simulink model "sim_TCC_2024"  (R2024b)
settings: Solver=FixedStepAuto  StartTime=0.0  StopTime=Tsim  FixedStep=Ts_sim  RelTol=1e-3
InitFcn:
  | traj
values from neighbouring files (symbols this model uses):
  dist = 0.1 * Lim_Torque_motor * [1, 1, 1]    [main_automacao.m]    (also in main_run.m = [0.5*Lim_Torque_motor,0.5*Lim_Torque_motor,0.5*Lim_Torque_mo)
  DISTURBANCE_ON = 1    [main_automacao.m]    (also in main_run.m)
  end_learning_time = 5 * Tspan    (= 50)    [main_automacao.m]    (also in main_run.m)
  error_difference = [ ... (first row only)    [main_automacao.m]    (also in main_run.m = [r(1),0,r(2),0,r(3),0])
  IC_ERROR_ON = 1    [main_automacao.m]    (also in main_run.m = 0)
  ILC_ON = method.ILC_ON    [main_automacao.m]    (also in main_run.m = 1)
  Kp0 = gains(1)    [main_automacao.m]    (also in main_run.m = 30)
  Kp1 = gains(3)    [main_automacao.m]    (also in main_run.m = 30)
  Kp2 = gains(5)    [main_automacao.m]    (also in main_run.m = 30)
  Kv0 = gains(2)    [main_automacao.m]    (also in main_run.m = 2.5)
  Kv1 = gains(4)    [main_automacao.m]    (also in main_run.m = 2.5)
  Kv2 = gains(6)    [main_automacao.m]    (also in main_run.m = 2.5)
  Lim_Torque_motor = 1.4    [main_automacao.m]    (also in main_run.m = 1)
  m_payload = 0.125    [main_automacao.m]    (also in main_run.m)
  NOISE_ON = 1    [main_automacao.m]    (also in main_run.m = 0)
  noise_power = [ ... (first row only)    [main_automacao.m]    (also in main_run.m = [1e-10,1e-10,1e-10,1e-10,1e-10,1e-10])
  PAYLOAD_ON = 1    [main_automacao.m]    (also in main_run.m = 0)
  SATURATION_ON = 1    [main_automacao.m]    (also in main_run.m)
  shift_time = Tspan / 2    (= 5)    [main_automacao.m]    (also in main_run.m; plot_trajetorias.m)
  t0_dist = end_learning_time + 2    (= 52)    [main_automacao.m]    (also in main_run.m = 26)
  t_pick = 0:Ts:Tspan/2-Ts    [main_automacao.m]    (also in main_run.m; plot_trajetorias.m = 0:Ts:cycle_duration/2-Ts)
  t_return = 0:Ts:Tspan/2-Ts    [main_automacao.m]    (also in main_run.m; plot_trajetorias.m = 0:Ts:cycle_duration/2-Ts)
  tf_dist = t0_dist + 2    (= 54)    [main_automacao.m]    (also in main_run.m = 32)
  Ts = 0.01    [main_automacao.m]    (also in main_run.m; plot_trajetorias.m)
  Tspan = 10    [main_automacao.m]    (also in main_run.m)
undefined symbols (not defined in the file or in its folder): q0_ida, q1_ida, q2_ida, qd0_ida, qd1_ida, qd2_ida, qdd0_ida, qdd1_ida, qdd2_ida
libraries: simulink x23, simulink_extras x3
settings Model: Creator=iury  LastModifiedBy=gabri
settings SolverCC: AlgebraicLoopSolver=TrustRegion
settings DataIOCC: ReturnWorkspaceOutputs=off
settings DebuggingCC: UnconnectedInputMsg=warning  UnconnectedOutputMsg=warning  UnconnectedLineMsg=warning  ArithmeticOperatorsInVariantConditions=warning
settings ModelReferenceCC: EnableRefExpFcnMdlSchedulingChecks=on
settings SFSimCC: SimUseLocalCustomCode=off  CustomCodeUndefinedFunction=UseInterfaceOnly
settings RTWCC: RTWUseLocalCustomCode=off  GPUComputeCapability=3.5
settings CodeAppCC: StateflowObjectComments=on
settings SimscapeCC: SimscapeNormalizeSystem=off

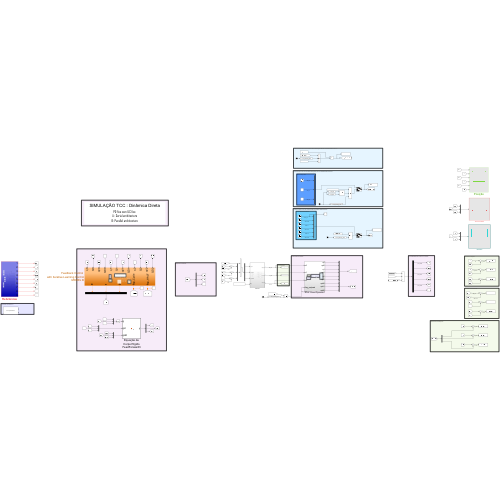
[thumbnail: Simulink's stored preview of the top-level diagram]
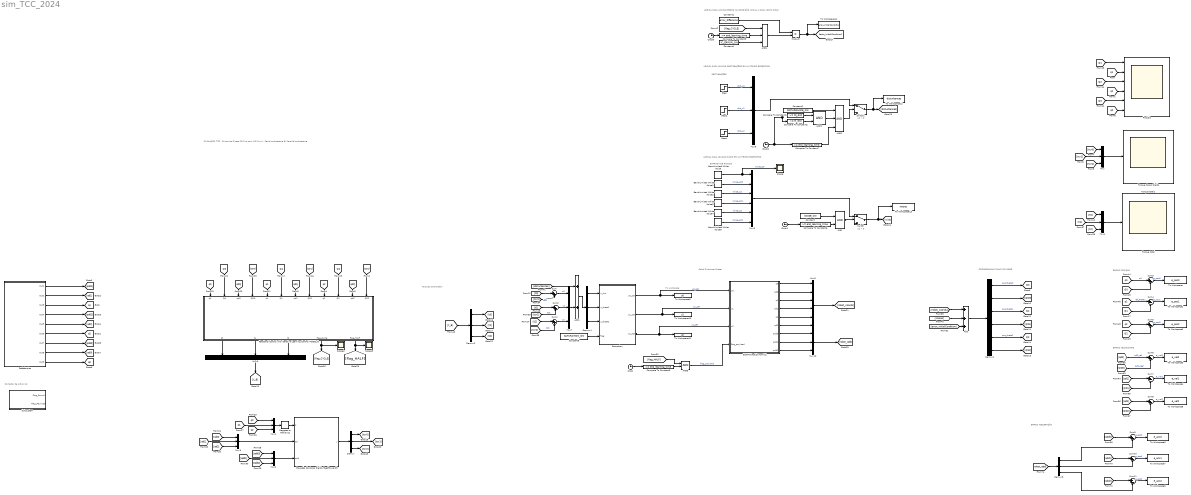
== system sim_TCC_2024 ==
  note: LÓGICA PARA APLICAR ERROS NA CONDIÇÃO INICIAL A CADA NOVO CICLO
  note: Contador de ciclos ILC
  note: PERTUBAÇÕES
  note: Torques controlador
  note: LÓGICA PARA APLICAR PERTUBAÇÕES EM UM TEMPO ESPECÍFICO
  note: Robô Dinâmica Direta
  note: COORDENADAS FINAIS DO ROBÔ
  note: ENTRADA DE RUÍDOS
  note: LÓGICA PARA APLICAR RUÍDO EM UM TEMPO ESPECÍFICO
  note: SIMULAÇÃO TCC : Dinâmica Direta
      |
      | PD fixo com ILC fixo
      | A : Serial architecture
      | B: Parallel architecture
  note: ERROS POSIÇAO
  note: ERROS VELOCIDADE
  note: ERROS ACELERAÇÃO
  note: To workspace
  3DOF Direct Dynamic1 : Subsystem
  AND : Logic  AllPortsSameDT=off  OutDataTypeStr=boolean
  AND1 : Logic  Inputs=3  AllPortsSameDT=off  OutDataTypeStr=boolean
  AND2 : Logic  AllPortsSameDT=off  OutDataTypeStr=boolean
  AND4 : Logic  Inputs=3  AllPortsSameDT=off  OutDataTypeStr=boolean
  AND5 : Logic  AllPortsSameDT=off  OutDataTypeStr=boolean
  Add : Sum  Inputs=+++
  Add1 : Sum
  Band-Limited White Noise : simulink/Sources/Band-Limited White Noise  Cov=noise_power(1)  Ts=Ts  seed=[1]
  Band-Limited White Noise1 : simulink/Sources/Band-Limited White Noise  Cov=noise_power(2)  Ts=Ts  seed=[2]
  Band-Limited White Noise2 : simulink/Sources/Band-Limited White Noise  Cov=noise_power(3)  Ts=Ts  seed=[3]
  Band-Limited White Noise3 : simulink/Sources/Band-Limited White Noise  Cov=noise_power(4)  Ts=Ts  seed=[4]
  Band-Limited White Noise4 : simulink/Sources/Band-Limited White Noise  Cov=noise_power(5)  Ts=Ts  seed=[5]
  Band-Limited White Noise5 : simulink/Sources/Band-Limited White Noise  Cov=noise_power(6)  Ts=Ts  seed=[6]
  Clock{,1..3} (4 alike) : Clock
  Compare To Constant1 : simulink/Logic and Bit Operations/Compare To Constant  relop=>=  const=t0_dist  OutDataTypeStr=boolean
  Compare To Constant2 : simulink/Logic and Bit Operations/Compare To Constant  relop=<=  const=tf_dist  OutDataTypeStr=boolean
  Compare To Constant{3,5..7} (4 alike) : simulink/Logic and Bit Operations/Compare To Constant  relop=>=  const=end_learning_time  OutDataTypeStr=boolean
  Constant : Constant  Value=NOISE_ON
  Constant1 : Constant  Value=error_difference
  Constant2 : Constant  Value=DISTURBANCE_ON
  Constant4 : Constant  Value=IC_ERROR_ON
  Constant5 : Constant  Value=SATURATION_ON
  Degrees to Radians2 : simulink_extras/Transformations/Degrees to Radians
  Demux{,2..4} (4 alike) : Demux  Outputs=3
  Demux1 : Demux  Outputs=6
  Equação de Corpo Rígido FeedForward3 : MATLAB Function  TreatAsAtomicUnit=on
  Feedback Control with Iterative Learning Control MODEL B : Subsystem
  Mux{,1..4,6..7,9..10} (9 alike) : Mux  Inputs=3
  Mux5 : Mux  Inputs=6
  Mux8 : Mux  Inputs=6
  Posição : Scope  NumInputPorts=6
  Product : Product
  Referências : Subsystem
  Saturation : Subsystem
  Scope : Scope
  Scope2 : Scope
  Scope3 : Scope
  Step : Step  After=dist(1)  SampleTime=Ts
  Step2 : Step  After=dist(2)  SampleTime=Ts
  Step4 : Step  After=dist(3)  SampleTime=Ts
  Subsystem : Subsystem  mask{Tspan=Tspan, Parameter3=Ts}
      mask prompts: Parameter3 "Sample Time"
      mask Display: disp('ILC Cycle Counter');
  Sum : Sum  Inputs=|++
  Sum1 : Sum  Inputs=|++
  Sum{3..11} (9 alike) : Sum  Inputs=|+-
  Sum2 : Sum  Inputs=|++
  Switch : Switch  Criteria=u2 > Threshold  SaturateOnIntegerOverflow=off  InputSameDT=off
  Switch1 : Switch  Criteria=u2 > Threshold  SaturateOnIntegerOverflow=off  InputSameDT=off
  To Workspace : ToWorkspace  VariableName=e_pos0  SaveFormat=Timeseries  SampleTime=-1
  To Workspace1 : ToWorkspace  VariableName=e_pos1  SaveFormat=Timeseries  SampleTime=-1
  To Workspace10 : ToWorkspace  VariableName=u1  SaveFormat=Timeseries  SampleTime=-1
  To Workspace11 : ToWorkspace  VariableName=u2  SaveFormat=Timeseries  SampleTime=-1
  To Workspace12 : ToWorkspace  VariableName=disturbances  SaveFormat=Timeseries  SampleTime=-1
  To Workspace13 : ToWorkspace  VariableName=noises  SaveFormat=Timeseries  SampleTime=-1
  To Workspace14 : ToWorkspace  VariableName=error_initialCondition  SaveFormat=Timeseries  SampleTime=-1
  To Workspace2 : ToWorkspace  VariableName=e_pos2  SaveFormat=Timeseries  SampleTime=-1
  To Workspace3 : ToWorkspace  VariableName=e_vel0  SaveFormat=Timeseries  SampleTime=-1
  To Workspace4 : ToWorkspace  VariableName=e_vel1  SaveFormat=Timeseries  SampleTime=-1
  To Workspace5 : ToWorkspace  VariableName=e_vel2  SaveFormat=Timeseries  SampleTime=-1
  To Workspace6 : ToWorkspace  VariableName=e_acc0  SaveFormat=Timeseries  SampleTime=-1
  To Workspace7 : ToWorkspace  VariableName=e_acc1  SaveFormat=Timeseries  SampleTime=-1
  To Workspace8 : ToWorkspace  VariableName=e_acc2  SaveFormat=Timeseries  SampleTime=-1
  To Workspace9 : ToWorkspace  VariableName=u0  SaveFormat=Timeseries  SampleTime=-1
  Torque Corpo Rígido : Scope
  Torque total : Scope
  Torque total1 : Scope
  tag scope: Q0=global, Q1=global, Q2=global, q0=global, q1=global, q2=global
  wires:
  Mux/1 -> Torque Corpo Rígido/1
  [q0] -> Feedback Control with Iterative Learning Control MODEL B/1(q0)
  [Q0] -> Feedback Control with Iterative Learning Control MODEL B/2(Q0)
  [qd0] -> Feedback Control with Iterative Learning Control MODEL B/3(qd0)
  [QD0] -> Feedback Control with Iterative Learning Control MODEL B/4(QD0)
  [q1] -> Feedback Control with Iterative Learning Control MODEL B/5(q1)
  [Q1] -> Feedback Control with Iterative Learning Control MODEL B/6(Q1)
  [qd1] -> Feedback Control with Iterative Learning Control MODEL B/7(qd1)
  [QD1] -> Feedback Control with Iterative Learning Control MODEL B/8(QD1)
  [q2] -> Feedback Control with Iterative Learning Control MODEL B/9(q2)
  [Q2] -> Feedback Control with Iterative Learning Control MODEL B/10(Q2)
  [QD2] -> Feedback Control with Iterative Learning Control MODEL B/12(QD2)
  [qd2] -> Feedback Control with Iterative Learning Control MODEL B/11(qd2)
  [Q1] -> Posição/1
  [q1] -> Posição/2
  [Q2] -> Posição/3
  [q2] -> Posição/4
  [Q0] -> Posição/5
  [q0] -> Posição/6
  Mux1/1 -> Degrees to Radians2/1
  [q0] -> Mux1/1
  [q2] -> Mux1/3
  [q1] -> Mux1/2
  [qdd0] -> Mux2/1
  [qdd2] -> Mux2/3
  [qdd1] -> Mux2/2
  [qd2] -> Mux3/3
  [qd1] -> Mux3/2
  [qd0] -> Mux3/1
  Demux/1 -> [tcr0]
  Demux/3 -> [tcr2]
  Demux/2 -> [tcr1]
  Equação de Corpo Rígido FeedForward3/1(y) -> Demux/1
  Mux3/1 -> Equação de Corpo Rígido FeedForward3/2(qd)
  Mux2/1 -> Equação de Corpo Rígido FeedForward3/3(qdd)
  Degrees to Radians2/1 -> Equação de Corpo Rígido FeedForward3/1(q)
  [tcr0] -> Mux/1
  [tcr1] -> Mux/2
  [tcr2] -> Mux/3
  [t1] -> Mux4/2
  Mux4/1 -> Torque total/1
  [t2] -> Mux4/3
  [t0] -> Mux4/1
  Feedback Control with Iterative Learning Control MODEL B/2(t1) -> Mux9/2
  Feedback Control with Iterative Learning Control MODEL B/3(t2) -> Mux9/3
  Feedback Control with Iterative Learning Control MODEL B/1(t0) -> Mux9/1
  [t0] -> Sum/1
  [t2] -> Sum1/1
  [t1] -> Sum2/1
  [tcr0] -> Sum/2  "tcr0"
  [tcr2] -> Sum1/2  "tcr2"
  [tcr1] -> Sum2/2  "tcr1"
  Band-Limited White Noise/1 -> Scope/1, Mux5/1  "noise_q0"
  Band-Limited White Noise1/1 -> Mux5/2  "noise_qd0"
  Band-Limited White Noise2/1 -> Mux5/3  "noise_q1"
  Band-Limited White Noise3/1 -> Mux5/4  "noise_qd1"
  Band-Limited White Noise4/1 -> Mux5/5  "noise_q2"
  Band-Limited White Noise5/1 -> Mux5/6  "noise_qd2"
  Mux5/1 -> Switch/1
  Demux1/1 -> [Q0]  "pos_theta0"
  Demux1/2 -> [QD0]
  Demux1/3 -> [Q1]  "pos_theta1"
  Demux1/4 -> [QD1]
  Demux1/5 -> [Q2]  "pos_theta2"
  Demux1/6 -> [QD2]
  Add/1 -> Demux1/1
  Constant/1 -> AND/1
  AND/1 -> Switch/2
  3DOF Direct Dynamic1/1(q0) -> Mux8/1
  3DOF Direct Dynamic1/2(qd0) -> Mux8/2
  3DOF Direct Dynamic1/3(q1) -> Mux8/3
  3DOF Direct Dynamic1/4(qd1) -> Mux8/4
  3DOF Direct Dynamic1/5(q2) -> Mux8/5
  3DOF Direct Dynamic1/6(qd2) -> Mux8/6
  Step/1 -> Mux6/1  "dist_u0"
  Step2/1 -> Mux6/2  "dist_u1"
  Step4/1 -> Mux6/3  "dist_u2"
  AND1/1 -> Switch1/2
  Constant2/1 -> AND1/1
  Compare To Constant1/1 -> AND2/1
  Compare To Constant2/1 -> AND2/2
  Clock2/1 -> Compare To Constant2/1, Compare To Constant1/1, Compare To Constant7/1
  Mux6/1 -> Switch1/1
  Switch1/1 -> To Workspace12/1, [disturbances]
  Switch/1 -> To Workspace13/1, [noises]
  Mux9/1 -> [t_B]
  [t_B] -> Demux2/1
  Demux2/1 -> [t0]
  Demux2/2 -> [t1]
  Demux2/3 -> [t2]
  [q0] -> Sum3/1  "q0"
  Sum3/1 -> To Workspace/1  "e_pos0"
  [q2] -> Sum5/1
  [Q1] -> Sum4/2
  [Q2] -> Sum5/2
  [Q0] -> Sum3/2
  [q1] -> Sum4/1  "ref_theta1"
  Sum4/1 -> To Workspace1/1  "e_pos1"
  Sum5/1 -> To Workspace2/1  "e_pos2"
  Sum7/1 -> To Workspace4/1  "e_vel1"
  [QD1] -> Sum7/2
  [qd1] -> Sum7/1
  [qd0] -> Sum6/1  "qd0_ref"
  [QD2] -> Sum8/2
  Sum6/1 -> To Workspace3/1  "e_vel0"
  [qd2] -> Sum8/1
  [QD0] -> Sum6/2  "qd0_real"
  Sum8/1 -> To Workspace5/1  "e_vel2"
  Sum10/1 -> To Workspace7/1  "e_acc1"
  [qdd1] -> Sum10/1
  Sum11/1 -> To Workspace8/1  "e_acc2"
  [qdd0] -> Sum9/1
  Demux3/2 -> Sum10/2
  Demux3/1 -> Sum9/2
  Sum9/1 -> To Workspace6/1  "e_acc0"
  Demux3/3 -> Sum11/2
  [qdd2] -> Sum11/1
  3DOF Direct Dynamic1/7(qdd0) -> Mux10/1
  3DOF Direct Dynamic1/8(qdd1) -> Mux10/2
  3DOF Direct Dynamic1/9(qdd2) -> Mux10/3
  Mux10/1 -> [robot_qdd]
  [robot_qdd] -> Demux3/1
  [robot_coords] -> Add/1
  [noises] -> Add/2
  [flag_CYCLE] -> AND4/1
  [error_initialCondition] -> Add/3
  Constant4/1 -> AND4/3
  Referências/1(Out1) -> [qdd1]
  Referências/2(Out2) -> [qd1]
  Referências/3(Out3) -> [q1]
  Referências/4(Out4) -> [qdd2]
  Referências/5(Out5) -> [qd2]
  Referências/6(Out6) -> [q2]
  Referências/7(Out7) -> [qdd0]
  Referências/8(Out8) -> [qd0]
  Referências/9(Out9) -> [q0]
  Mux8/1 -> [robot_coords]
  Saturation/1(u0_sat) -> 3DOF Direct Dynamic1/1(u0), To Workspace9/1  "u0_sat"
  Saturation/2(u1_sat) -> To Workspace10/1, 3DOF Direct Dynamic1/2(u1)  "u1_sat"
  Saturation/3(u2_sat) -> 3DOF Direct Dynamic1/3(u2), To Workspace11/1  "u2_sat"
  Constant5/1 -> Saturation/4(flag)
  Sum2/1 -> Mux7/2  "u1"
  Sum/1 -> Mux7/1  "u0"
  Sum1/1 -> Mux7/3  "u2"
  [disturbances] -> Add1/1
  Mux7/1 -> Add1/2
  Add1/1 -> Demux4/1
  Demux4/1 -> Saturation/1(u_rho)
  Demux4/2 -> Saturation/2(u_theta1)
  Demux4/3 -> Saturation/3(u_theta2)
  AND2/1 -> AND1/2
  [flag_HALF] -> AND5/1
  AND5/1 -> 3DOF Direct Dynamic1/4(flag_payload)  "flag_payload"
  Clock/1 -> Compare To Constant5/1
  Compare To Constant5/1 -> AND5/2
  Feedback Control with Iterative Learning Control MODEL B/4(flag_Cycle) -> Scope2/1, [flag_CYCLE]
  Feedback Control with Iterative Learning Control MODEL B/5(flag_HALF) -> Scope3/1, [flag_HALF]
  Clock1/1 -> Compare To Constant6/1
  Compare To Constant6/1 -> AND/2
  Compare To Constant7/1 -> AND1/3
  Compare To Constant3/1 -> AND4/2
  Clock3/1 -> Compare To Constant3/1
  AND4/1 -> Product/2
  Constant1/1 -> Product/1
  Product/1 -> To Workspace14/1, [error_initialCondition]

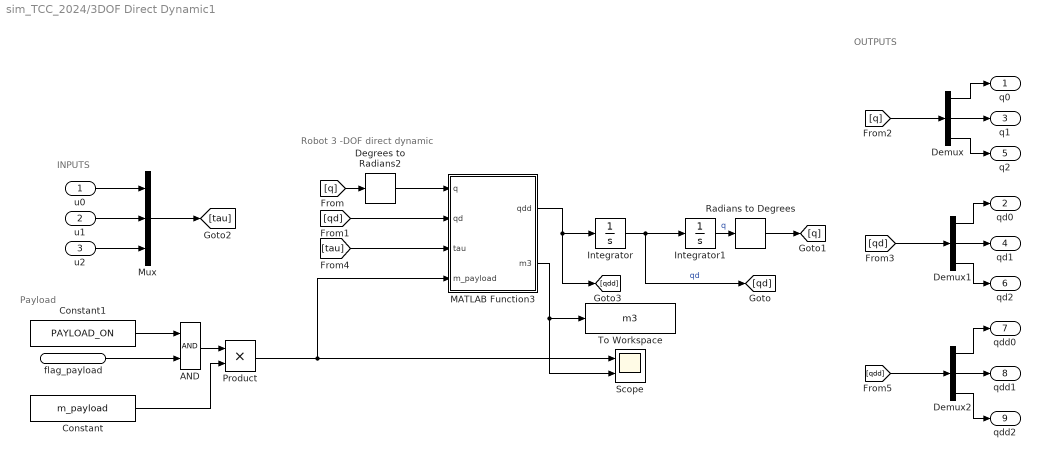
== system sim_TCC_2024/3DOF Direct Dynamic1 ==
  note: Payload
  note: INPUTS
  note: Robot 3 -DOF direct dynamic
  note: OUTPUTS
  u0 : Inport
  u1 : Inport  Port=2
  u2 : Inport  Port=3
  flag_payload : Inport  Port=4
  AND : Logic  AllPortsSameDT=off  OutDataTypeStr=boolean
  Constant : Constant  Value=m_payload
  Constant1 : Constant  Value=PAYLOAD_ON
  Degrees to Radians2 : simulink_extras/Transformations/Degrees to Radians
  Demux : Demux  Outputs=3
  Demux1 : Demux  Outputs=3
  Demux2 : Demux  Outputs=3
  Integrator : Integrator  InitialCondition=[0;0;0]
  Integrator1 : Integrator  InitialCondition=[0;0;0]
  MATLAB Function3 : MATLAB Function  TreatAsAtomicUnit=on
  Mux : Mux  Inputs=3
  Product : Product
  Radians to Degrees : simulink_extras/Transformations/Radians to Degrees
  Scope : Scope  NumInputPorts=2
  To Workspace : ToWorkspace  VariableName=m3  SaveFormat=Timeseries  SampleTime=-1
  q0 : Outport
  qd0 : Outport  Port=2
  q1 : Outport  Port=3
  qd1 : Outport  Port=4
  q2 : Outport  Port=5
  qd2 : Outport  Port=6
  qdd0 : Outport  Port=7
  qdd1 : Outport  Port=8
  qdd2 : Outport  Port=9
  wires:
  Integrator/1 -> [qd], Integrator1/1  "qd"
  [q] -> Degrees to Radians2/1
  [qd] -> MATLAB Function3/2(qd)
  [q] -> Demux/1
  Demux/1 -> q0/1
  Demux/2 -> q1/1
  Demux/3 -> q2/1
  [qd] -> Demux1/1
  Demux1/1 -> qd0/1
  Demux1/2 -> qd1/1
  Demux1/3 -> qd2/1
  [tau] -> MATLAB Function3/3(tau)
  u0/1 -> Mux/1
  u1/1 -> Mux/2
  u2/1 -> Mux/3
  Mux/1 -> [tau]
  Integrator1/1 -> Radians to Degrees/1  "q"
  Radians to Degrees/1 -> [q]
  MATLAB Function3/1(qdd) -> [qdd], Integrator/1
  [qdd] -> Demux2/1
  Demux2/1 -> qdd0/1
  Demux2/2 -> qdd1/1
  Demux2/3 -> qdd2/1
  Constant1/1 -> AND/1
  flag_payload/1 -> AND/2
  MATLAB Function3/2(m3) -> Scope/2, To Workspace/1
  AND/1 -> Product/1
  Constant/1 -> Product/2
  Product/1 -> Scope/1, MATLAB Function3/4(m_payload)
  Degrees to Radians2/1 -> MATLAB Function3/1(q)

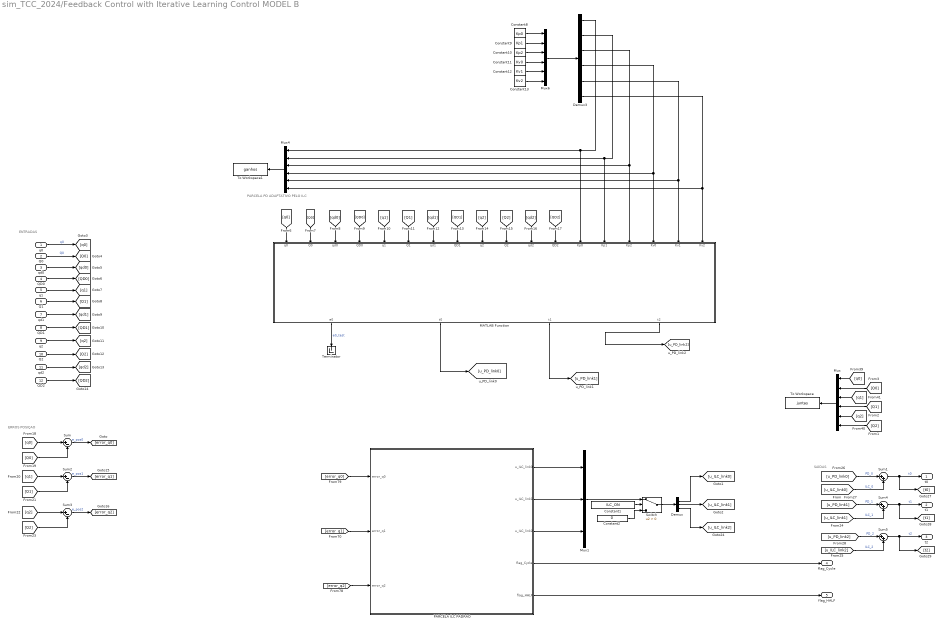
== system sim_TCC_2024/Feedback Control with Iterative Learning Control MODEL B ==
  note: PARCELA PD ADAPTATIVO PELO ILC
  note: SAÍDAS
  note: ERROS POSIÇAO
  note: ENTRADAS
  q0 : Inport
  Q0 : Inport  Port=2
  qd0 : Inport  Port=3
  QD0 : Inport  Port=4
  q1 : Inport  Port=5
  Q1 : Inport  Port=6
  qd1 : Inport  Port=7
  QD1 : Inport  Port=8
  q2 : Inport  Port=9
  Q2 : Inport  Port=10
  qd2 : Inport  Port=11
  QD2 : Inport  Port=12
  Constant1 : Constant  Value=ILC_ON
  Constant10 : Constant  Value=Kp2
  Constant11 : Constant  Value=Kv0
  Constant12 : Constant  Value=Kv1
  Constant13 : Constant  Value=Kv2
  Constant2 : Constant  Value=0
  Constant8 : Constant  Value=Kp0
  Constant9 : Constant  Value=Kp1
  Demux : Demux  Outputs=3
  Demux3 : Demux  Outputs=6
  MATLAB Function : MATLAB Function  TreatAsAtomicUnit=on
  Mux : Mux  Inputs=6
  Mux1 : Mux  Inputs=3
  Mux4 : Mux  Inputs=6
  Mux6 : Mux  Inputs=6
  PARCELA ILC PADRAO : Subsystem
  Sum : Sum  Inputs=|+-
  Sum1 : Sum  Inputs=|++
  Sum2 : Sum  Inputs=|+-
  Sum3 : Sum  Inputs=|+-
  Sum4 : Sum  Inputs=|++
  Sum5 : Sum  Inputs=|++
  Switch : Switch  Criteria=u2 > Threshold  SaturateOnIntegerOverflow=off  InputSameDT=off
  Terminator : Terminator
  To Workspace : ToWorkspace  VariableName=juntas  SaveFormat=Timeseries  SampleTime=-1
  To Workspace1 : ToWorkspace  VariableName=ganhos  SaveFormat=Timeseries  SampleTime=-1
  t0 : Outport
  t1 : Outport  Port=2
  t2 : Outport  Port=3
  flag_Cycle : Outport  Port=4
  flag_HALF : Outport  Port=5
  wires:
  Mux/1 -> To Workspace/1
  [q0] -> Mux/1
  [q1] -> Mux/3
  [q2] -> Mux/5
  [Q2] -> Mux/6
  [Q1] -> Mux/4
  [Q0] -> Mux/2
  Mux4/1 -> To Workspace1/1
  Sum/1 -> [error_q0]  "e_pos0"
  MATLAB Function/2(t0) -> [u_PD_link0]
  q0/1 -> [q0]  "q0"
  Q0/1 -> [Q0]  "Q0"
  qd0/1 -> [qd0]
  QD0/1 -> [QD0]
  q1/1 -> [q1]
  Q1/1 -> [Q1]
  qd1/1 -> [qd1]
  QD1/1 -> [QD1]
  q2/1 -> [q2]
  Q2/1 -> [Q2]
  qd2/1 -> [qd2]
  QD2/1 -> [QD2]
  [q0] -> MATLAB Function/1(q0)
  [Q0] -> MATLAB Function/2(Q0)
  [qd0] -> MATLAB Function/3(qd0)
  [QD0] -> MATLAB Function/4(QD0)
  [q1] -> MATLAB Function/5(q1)
  [Q1] -> MATLAB Function/6(Q1)
  [qd1] -> MATLAB Function/7(qd1)
  [QD1] -> MATLAB Function/8(QD1)
  [q2] -> MATLAB Function/9(q2)
  [Q2] -> MATLAB Function/10(Q2)
  [qd2] -> MATLAB Function/11(qd2)
  [QD2] -> MATLAB Function/12(QD2)
  [q0] -> Sum/1
  [Q0] -> Sum/2
  [Q1] -> Sum2/2
  [q1] -> Sum2/1
  Sum2/1 -> [error_q1]  "e_pos1"
  [Q2] -> Sum3/2
  [q2] -> Sum3/1
  Sum3/1 -> [error_q2]  "e_pos2"
  MATLAB Function/3(t1) -> [u_PD_link1]
  MATLAB Function/4(t2) -> [u_PD_link2]
  Sum1/1 -> [t0], t0/1  "t0"
  Sum4/1 -> [t1], t1/1  "t1"
  Sum5/1 -> [t2], t2/1  "t2"
  [u_ILC_link0] -> Sum1/2  "ILC_0"
  [u_ILC_link1] -> Sum4/2  "ILC_1"
  [u_ILC_link2] -> Sum5/2  "ILC_2"
  [u_PD_link1] -> Sum4/1  "PD_1"
  [u_PD_link2] -> Sum5/1  "PD_2"
  [u_PD_link0] -> Sum1/1  "PD_0"
  Constant8/1 -> Mux6/1
  Constant9/1 -> Mux6/2
  Constant10/1 -> Mux6/3
  Constant11/1 -> Mux6/4
  Constant12/1 -> Mux6/5
  Constant13/1 -> Mux6/6
  Demux3/1 -> MATLAB Function/13(Kp0), Mux4/1
  Demux3/2 -> MATLAB Function/14(Kp1), Mux4/2
  Demux3/3 -> Mux4/3, MATLAB Function/15(Kp2)
  Demux3/4 -> Mux4/4, MATLAB Function/16(Kv0)
  Demux3/6 -> MATLAB Function/18(Kv2), Mux4/6
  Demux3/5 -> Mux4/5, MATLAB Function/17(Kv1)
  [error_q2] -> PARCELA ILC PADRAO/3(error_q2)
  [error_q1] -> PARCELA ILC PADRAO/2(error_q1)
  [error_q0] -> PARCELA ILC PADRAO/1(error_q0)
  Mux6/1 -> Demux3/1
  MATLAB Function/1(e0) -> Terminator/1  "e0_test"
  Constant1/1 -> Switch/2
  Mux1/1 -> Switch/1
  PARCELA ILC PADRAO/3(u_ILC_link2) -> Mux1/3
  PARCELA ILC PADRAO/2(u_ILC_link1) -> Mux1/2
  PARCELA ILC PADRAO/1(u_ILC_link0) -> Mux1/1
  Switch/1 -> Demux/1
  Demux/1 -> [u_ILC_link0]
  Demux/2 -> [u_ILC_link1]
  Demux/3 -> [u_ILC_link2]
  Constant2/1 -> Switch/3
  PARCELA ILC PADRAO/4(flag_Cycle) -> flag_Cycle/1
  PARCELA ILC PADRAO/5(flag_HALF) -> flag_HALF/1

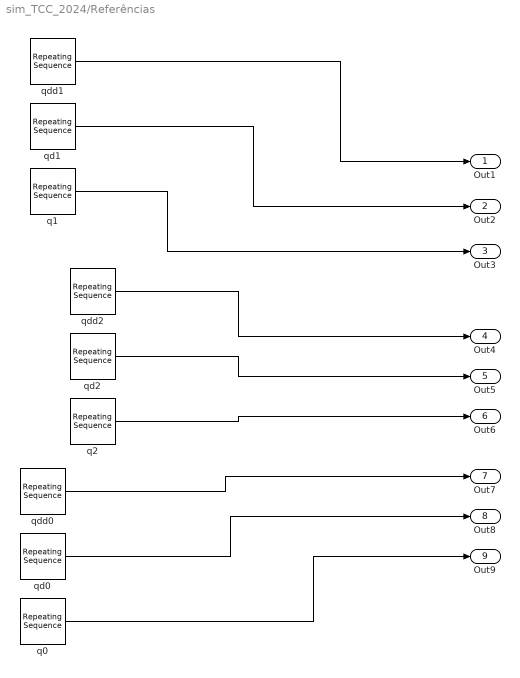
== system sim_TCC_2024/Referências ==
  q0 : simulink/Sources/Repeating Sequence  rep_seq_t=[t_pick (t_return+shift_time) ]  rep_seq_y=[q0_ida(:,2)' q0_volta(:,2)' ]
  q1 : simulink/Sources/Repeating Sequence  rep_seq_t=[t_pick (t_return+shift_time) ]  rep_seq_y=[q1_ida(:,2)' q1_volta(:,2)' ]
  q2 : simulink/Sources/Repeating Sequence  rep_seq_t=[t_pick (t_return+shift_time) ]  rep_seq_y=[q2_ida(:,2)' q2_volta(:,2)' ]
  qd0 : simulink/Sources/Repeating Sequence  rep_seq_t=[t_pick (t_return+shift_time)]  rep_seq_y=[qd0_ida(:,2)' qd0_volta(:,2)' ]
  qd1 : simulink/Sources/Repeating Sequence  rep_seq_t=[t_pick (t_return+shift_time)]  rep_seq_y=[qd1_ida(:,2)' qd1_volta(:,2)']
  qd2 : simulink/Sources/Repeating Sequence  rep_seq_t=[t_pick (t_return+shift_time) ]  rep_seq_y=[qd2_ida(:,2)' qd2_volta(:,2)' ]
  qdd0 : simulink/Sources/Repeating Sequence  rep_seq_t=[t_pick (t_return+shift_time) ]  rep_seq_y=[qdd0_ida(:,2)' qdd0_volta(:,2)' ]
  qdd1 : simulink/Sources/Repeating Sequence  rep_seq_t=[t_pick , (t_return+shift_time)]  rep_seq_y=[qdd1_ida(:,2)' ,qdd1_volta(:,2)' ]
  qdd2 : simulink/Sources/Repeating Sequence  rep_seq_t=[t_pick (t_return+shift_time)]  rep_seq_y=[qdd2_ida(:,2)' qdd2_volta(:,2)' ]
  Out1 : Outport
  Out2 : Outport  Port=2
  Out3 : Outport  Port=3
  Out4 : Outport  Port=4
  Out5 : Outport  Port=5
  Out6 : Outport  Port=6
  Out7 : Outport  Port=7
  Out8 : Outport  Port=8
  Out9 : Outport  Port=9
  wires:
  qdd1/1 -> Out1/1
  qd1/1 -> Out2/1
  q1/1 -> Out3/1
  qdd2/1 -> Out4/1
  qd2/1 -> Out5/1
  q2/1 -> Out6/1
  qdd0/1 -> Out7/1
  qd0/1 -> Out8/1
  q0/1 -> Out9/1

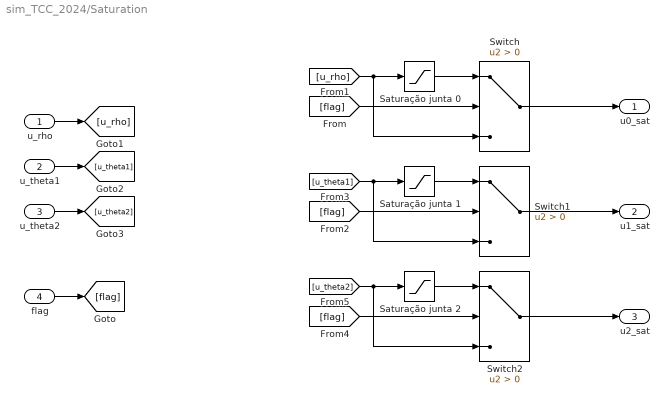
== system sim_TCC_2024/Saturation ==
  u_rho : Inport
  u_theta1 : Inport  Port=2
  u_theta2 : Inport  Port=3
  flag : Inport  Port=4
  Saturação junta 0 : Saturate  UpperLimit=Lim_Torque_motor  LowerLimit=-Lim_Torque_motor
  Saturação junta 1 : Saturate  UpperLimit=Lim_Torque_motor  LowerLimit=-Lim_Torque_motor
  Saturação junta 2 : Saturate  UpperLimit=Lim_Torque_motor  LowerLimit=-Lim_Torque_motor
  Switch : Switch  Criteria=u2 > Threshold  SaturateOnIntegerOverflow=off  InputSameDT=off
  Switch1 : Switch  Criteria=u2 > Threshold  SaturateOnIntegerOverflow=off  InputSameDT=off
  Switch2 : Switch  Criteria=u2 > Threshold  SaturateOnIntegerOverflow=off  InputSameDT=off
  u0_sat : Outport
  u1_sat : Outport  Port=2
  u2_sat : Outport  Port=3
  wires:
  Saturação junta 0/1 -> Switch/1
  flag/1 -> [flag]
  [flag] -> Switch/2
  u_rho/1 -> [u_rho]
  u_theta1/1 -> [u_theta1]
  u_theta2/1 -> [u_theta2]
  [u_rho] -> Switch/3, Saturação junta 0/1
  [flag] -> Switch1/2
  [u_theta1] -> Switch1/3, Saturação junta 1/1
  Saturação junta 1/1 -> Switch1/1
  [flag] -> Switch2/2
  [u_theta2] -> Switch2/3, Saturação junta 2/1
  Saturação junta 2/1 -> Switch2/1
  Switch/1 -> u0_sat/1
  Switch2/1 -> u2_sat/1
  Switch1/1 -> u1_sat/1

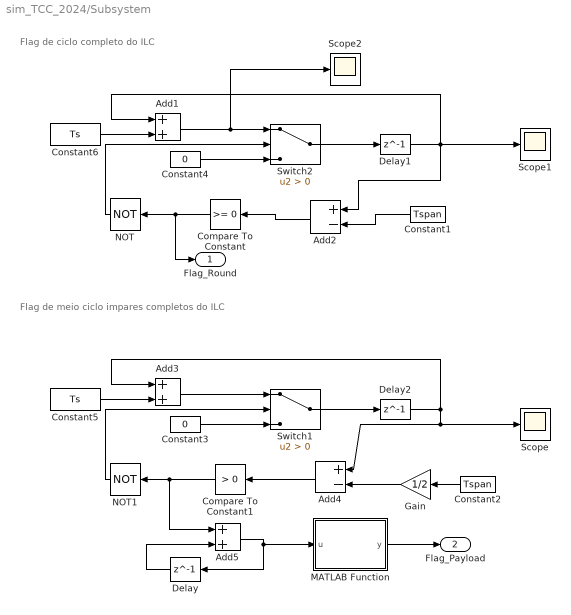
== system sim_TCC_2024/Subsystem ==
  note: Flag de ciclo completo do ILC
  note: Flag de meio ciclo impares completos do ILC
  Add1 : Sum
  Add2 : Sum  Inputs=+-
  Add3 : Sum
  Add4 : Sum  Inputs=+-
  Add5 : Sum
  Compare To Constant : simulink/Logic and Bit Operations/Compare To Constant  relop=>=  const=0  OutDataTypeStr=boolean
  Compare To Constant1 : simulink/Logic and Bit Operations/Compare To Constant  relop=>  const=0  OutDataTypeStr=uint8
  Constant1 : Constant  Value=Tspan
  Constant2 : Constant  Value=Tspan
  Constant3 : Constant  Value=0
  Constant4 : Constant  Value=0
  Constant5 : Constant  Value=Ts  SampleTime=Ts
  Constant6 : Constant  Value=Ts  SampleTime=Ts
  Delay : Delay  DelayLength=1  SampleTime=Ts
  Delay1 : Delay  DelayLength=1  InitialCondition=0  SampleTime=Ts
  Delay2 : Delay  DelayLength=1  InitialCondition=0  SampleTime=Ts
  Gain : Gain  Gain=1/2
  MATLAB Function : MATLAB Function  TreatAsAtomicUnit=on  SystemSampleTime=Ts
  NOT : Logic  Operator=NOT  AllPortsSameDT=off  OutDataTypeStr=boolean
  NOT1 : Logic  Operator=NOT  AllPortsSameDT=off  OutDataTypeStr=boolean
  Scope : Scope
  Scope1 : Scope
  Scope2 : Scope
  Switch1 : Switch  Criteria=u2 > Threshold  SaturateOnIntegerOverflow=off  InputSameDT=off
  Switch2 : Switch  Criteria=u2 > Threshold  SaturateOnIntegerOverflow=off  InputSameDT=off
  Flag_Round : Outport
  Flag_Payload : Outport  Port=2
  wires:
  Constant1/1 -> Add2/2
  Delay1/1 -> Add1/1, Scope1/1, Add2/1
  Switch2/1 -> Delay1/1
  Constant4/1 -> Switch2/3
  Add1/1 -> Scope2/1, Switch2/1
  NOT/1 -> Switch2/2
  Add2/1 -> Compare To Constant/1
  Constant6/1 -> Add1/2
  Compare To Constant/1 -> Flag_Round/1, NOT/1
  Add3/1 -> Switch1/1
  Constant2/1 -> Gain/1
  NOT1/1 -> Switch1/2
  Switch1/1 -> Delay2/1
  Constant5/1 -> Add3/2
  Delay2/1 -> Add3/1, Add4/1, Scope/1
  Add4/1 -> Compare To Constant1/1
  Constant3/1 -> Switch1/3
  Compare To Constant1/1 -> NOT1/1, Add5/1
  Gain/1 -> Add4/2
  Add5/1 -> MATLAB Function/1(u), Delay/1
  MATLAB Function/1(y) -> Flag_Payload/1
  Delay/1 -> Add5/2

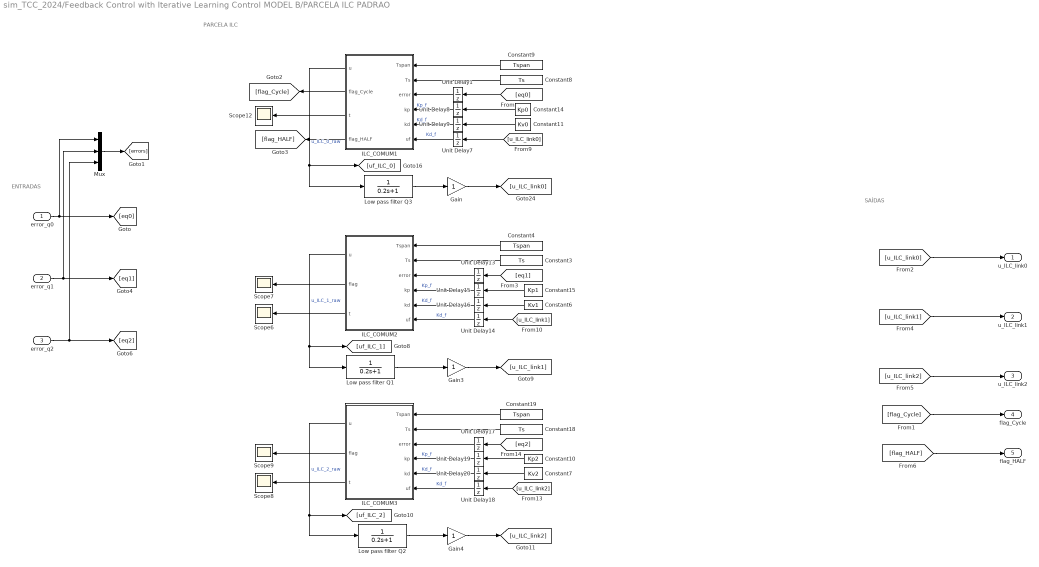
== system sim_TCC_2024/Feedback Control with Iterative Learning Control MODEL B/PARCELA ILC PADRAO ==
  note: SAÍDAS
  note: ENTRADAS
  note: PARCELA ILC
  error_q0 : Inport
  error_q1 : Inport  Port=2
  error_q2 : Inport  Port=3
  Constant10 : Constant  Value=Kp2
  Constant11 : Constant  Value=Kv0
  Constant14 : Constant  Value=Kp0
  Constant15 : Constant  Value=Kp1
  Constant18 : Constant  Value=Ts
  Constant19 : Constant  Value=Tspan
  Constant3 : Constant  Value=Ts
  Constant4 : Constant  Value=Tspan
  Constant6 : Constant  Value=Kv1
  Constant7 : Constant  Value=Kv2
  Constant8 : Constant  Value=Ts
  Constant9 : Constant  Value=Tspan
  Gain : Gain
  Gain3 : Gain
  Gain4 : Gain
  ILC_COMUM1 : MATLAB Function  TreatAsAtomicUnit=on  SystemSampleTime=Ts
  ILC_COMUM2 : MATLAB Function  TreatAsAtomicUnit=on  SystemSampleTime=Ts
  ILC_COMUM3 : MATLAB Function  TreatAsAtomicUnit=on  SystemSampleTime=Ts
  Low pass filter Q1 : TransferFcn  Denominator=[0.2 1]
  Low pass filter Q2 : TransferFcn  Denominator=[0.2 1]
  Low pass filter Q3 : TransferFcn  Denominator=[0.2 1]
  Mux : Mux  Inputs=3
  Scope{6..9,12} (5 alike) : Scope
  Unit Delay1 : UnitDelay  SampleTime=Ts  HasFrameUpgradeWarning=on
  Unit Delay13 : UnitDelay  SampleTime=Ts  HasFrameUpgradeWarning=on
  Unit Delay{7,9,14,16,18,20} (6 alike) : UnitDelay  InitialCondition=2.5  SampleTime=Ts  HasFrameUpgradeWarning=on
  Unit Delay15 : UnitDelay  InitialCondition=30  SampleTime=Ts  HasFrameUpgradeWarning=on
  Unit Delay17 : UnitDelay  SampleTime=Ts  HasFrameUpgradeWarning=on
  Unit Delay19 : UnitDelay  InitialCondition=30  SampleTime=Ts  HasFrameUpgradeWarning=on
  Unit Delay8 : UnitDelay  InitialCondition=30  SampleTime=Ts  HasFrameUpgradeWarning=on
  u_ILC_link0 : Outport
  u_ILC_link1 : Outport  Port=2
  u_ILC_link2 : Outport  Port=3
  flag_Cycle : Outport  Port=4
  flag_HALF : Outport  Port=5
  wires:
  Constant14/1 -> Unit Delay8/1
  Gain/1 -> [u_ILC_link0]
  Unit Delay1/1 -> ILC_COMUM1/3(error)
  Constant11/1 -> Unit Delay9/1
  error_q0/1 -> Mux/1, [eq0]
  [eq0] -> Unit Delay1/1
  error_q1/1 -> Mux/2, [eq1]
  error_q2/1 -> Mux/3, [eq2]
  [u_ILC_link0] -> u_ILC_link0/1
  [u_ILC_link1] -> u_ILC_link1/1
  [u_ILC_link2] -> u_ILC_link2/1
  Low pass filter Q3/1 -> Gain/1
  Constant9/1 -> ILC_COMUM1/1(Tspan)
  Constant8/1 -> ILC_COMUM1/2(Ts)
  Unit Delay8/1 -> ILC_COMUM1/4(kp)  "Kp_f"
  Unit Delay9/1 -> ILC_COMUM1/5(kd)  "Kd_f"
  ILC_COMUM1/1(u) -> Low pass filter Q3/1, [uf_ILC_0]  "u_ILC_0_raw"
  [u_ILC_link0] -> Unit Delay7/1
  Unit Delay7/1 -> ILC_COMUM1/6(uf)  "Kd_f"
  ILC_COMUM1/3(t) -> Scope12/1
  ILC_COMUM1/2(flag_Cycle) -> [flag_Cycle]
  ILC_COMUM2/2(flag) -> Scope7/1
  ILC_COMUM2/3(t) -> Scope6/1
  Unit Delay14/1 -> ILC_COMUM2/6(uf)  "Kd_f"
  [u_ILC_link1] -> Unit Delay14/1
  ILC_COMUM2/1(u) -> Low pass filter Q1/1, [uf_ILC_1]  "u_ILC_1_raw"
  Unit Delay16/1 -> ILC_COMUM2/5(kd)  "Kd_f"
  Unit Delay15/1 -> ILC_COMUM2/4(kp)  "Kp_f"
  Constant3/1 -> ILC_COMUM2/2(Ts)
  Constant4/1 -> ILC_COMUM2/1(Tspan)
  Low pass filter Q1/1 -> Gain3/1
  [eq1] -> Unit Delay13/1
  Constant6/1 -> Unit Delay16/1
  Unit Delay13/1 -> ILC_COMUM2/3(error)
  Gain3/1 -> [u_ILC_link1]
  Constant15/1 -> Unit Delay15/1
  Gain4/1 -> [u_ILC_link2]
  Unit Delay17/1 -> ILC_COMUM3/3(error)
  [eq2] -> Unit Delay17/1
  Low pass filter Q2/1 -> Gain4/1
  Constant19/1 -> ILC_COMUM3/1(Tspan)
  Constant18/1 -> ILC_COMUM3/2(Ts)
  Unit Delay19/1 -> ILC_COMUM3/4(kp)  "Kp_f"
  Unit Delay20/1 -> ILC_COMUM3/5(kd)  "Kd_f"
  ILC_COMUM3/1(u) -> Low pass filter Q2/1, [uf_ILC_2]  "u_ILC_2_raw"
  [u_ILC_link2] -> Unit Delay18/1
  Unit Delay18/1 -> ILC_COMUM3/6(uf)  "Kd_f"
  ILC_COMUM3/3(t) -> Scope8/1
  ILC_COMUM3/2(flag) -> Scope9/1
  Mux/1 -> [errors]
  ILC_COMUM1/4(flag_HALF) -> [flag_HALF]
  [flag_Cycle] -> flag_Cycle/1
  [flag_HALF] -> flag_HALF/1
  Constant10/1 -> Unit Delay19/1
  Constant7/1 -> Unit Delay20/1

== matlab function sim_TCC_2024/Feedback Control with Iterative Learning Control MODEL B/PARCELA ILC PADRAO/ILC_COMUM3 ==
  data: Tspan input; Ts input; u output; error input; flag output; t output; kp input; kd input; uf input
function [u, flag, t] = fcn(Tspan, Ts, error, kp, kd, uf)
persistent N samples_per_iter 
if isempty(N)
    N = round(Tspan/Ts); 
    samples_per_iter = N;
end

% -------------------------------------------------------------
% Memória persistente entre iterações
% -------------------------------------------------------------
persistent u_curr       % Comando de controle da iteração atual
persistent u_next       % Comando de controle da próxima iteração
persistent error_memory % Histórico de erros da iteração atual
persistent u_memory     % Histórico de torques da iteração atual
persistent k_iter       % Índice da iteração (ciclo)
persistent t_step       % Passo de tempo atual (1 até N)

if isempty(k_iter)
    k_iter = 1; 
    u_curr = zeros(1, N); 
    u_next = zeros(1, N);
    error_memory = zeros(1, N);
    u_memory = zeros(1, N);
    t_step = 1;
end

% -------------------------------------------------------------
% Lógica de Execução e Gravação (Sem saltar índices)
% -------------------------------------------------------------
% Aplica o torque calculado para o passo atual
u = u_curr(t_step);

% Grava perfeitamente os dados nas posições corretas (incluindo o passo 1)
error_memory(t_step) = error;
u_memory(t_step) = uf;

flag = 0; % Por padrão, a flag de fim de ciclo é zero

% -------------------------------------------------------------
% Lógica de Aprendizagem (Executada exatamente no último ponto)
% -------------------------------------------------------------
if t_step == samples_per_iter
    
    e_k = error_memory;
    % Extrapolação suave: repete o último ponto em vez de colocar 0, evitando o degrau
    e_k1 = [error_memory(2:end), error_memory(end)];
    
    % Lei de atualização do ILC + PD Corrigida:
    % kp multiplica o erro atual (e_k). kd multiplica a derivada correta.
  u_next = u_memory + kp*e_k + kd*(e_k1 - e_k);
    % u_next = u_memory + kp/10*e_k;
    
    % Atualiza o perfil para o próximo ciclo
    u_curr = u_next; 
    k_iter = k_iter + 1; 
    
    t_step = 1; % Reseta o contador para começar o próximo ciclo no passo 1
    flag = 1;   % Ativa a flag indicando fim de iteração
else
    t_step = t_step + 1; % Avança para o próximo passo de tempo
end

t = t_step;
end

== matlab function sim_TCC_2024/Subsystem/MATLAB Function ==
  data: u input; y output
function y = fcn(u)

resto = rem(u, 2);

if resto == 0
    y = 0;
else
    y = 1;
end

== matlab function sim_TCC_2024/3DOF Direct Dynamic1/MATLAB Function3 ==
  data: q input; qdd output; qd input; tau input; m_payload input; m3 output
function [qdd, m3] = RobotDynamic(q, qd, tau, m_payload)

% Parâmetros
l1 = 0.15;
l2 = 0.255;
l3 = 0.199;

m1 = 0.200;
m2 = 0.07576;
m3 = 0.07192 + m_payload;

g = 9.8;

theta2 = q(2);
theta3 = q(3);

v1 = qd(1);
v2 = qd(2);
v3 = qd(3);

% =========================
% MATRIZ DE INÉRCIA M(q)
% =========================

M11 = (1/2)*m1*l1^2 ...
    + (1/3)*m2*l2^2*cos(theta2)^2 ...
    + (1/3)*m3*l3^2*cos(theta2 + theta3)^2 ...
    + m3*l2^2*cos(theta2)^2 ...
    + m3*l2*l3*cos(theta2)*cos(theta2 + theta3);

M22 = (1/3)*m2*l2^2 ...
    + (1/3)*m3*l3^2 ...
    + m3*l2^2 ...
    + m3*l2*l3*cos(theta3);

M23 = (1/3)*m3*l3^2 ...
    + 0.5*m3*l2*l3*cos(theta3);

M33 = (1/3)*m3*l3^2;

M = [M11   0     0;
     0     M22   M23;
     0     M23   M33];

% =========================
% VETOR CORIOLIS/CENTRÍFUGO
% =========================

C1 = ( ...
    -(1/3)*m2*l2^2*sin(2*theta2) ...
    - m3*l2^2*sin(2*theta2) ...
    -(1/3)*m3*l3^2*sin(2*(theta2 + theta3)) ...
    - m3*l2*l3*sin(2*theta2 + theta3) ...
    )*v2*v1 ...
    + ( ...
    -(1/3)*m3*l3^2*sin(2*(theta2 + theta3)) ...
    - m3*l2*l3*cos(theta2)*sin(theta2 + theta3) ...
    )*v3*v1;

C2 = (-m3*l2*l3*sin(theta3))*v2*v3 ...
    + (-0.5*m3*l2*l3*sin(theta3))*v3^2 ...
    + ( ...
    (1/6)*m2*l2^2*sin(2*theta2) ...
    + (1/6)*m3*l3^2*sin(2*(theta2 + theta3)) ...
    + 0.5*m3*l2^2*sin(2*theta2) ...
    + 0.5*m3*l2*l3*sin(2*theta2 + theta3) ...
    )*v1^2;

C3 = (0.5*m3*l2*l3*sin(theta3))*v2^2 ...
    + ( ...
    (1/6)*m3*l3^2*sin(2*(theta2 + theta3)) ...
    + 0.5*m3*l2*l3*cos(theta2)*sin(theta2 + theta3) ...
    )*v1^2;

C = [C1; C2; C3];

% =========================
% VETOR GRAVITACIONAL G(q)
% =========================

G1 = 0;

G2 = 0.5*m2*g*l2*cos(theta2) ...
    + m3*g*l2*cos(theta2) ...
    + 0.5*m3*g*l3*cos(theta2 + theta3);

G3 = 0.5*m3*g*l3*cos(theta2 + theta3);

G = [G1; G2; G3];

% =========================
% ATRITO
% =========================

% Atrito Suavizado 
B = [0.1; 0.1; 0.1]; 

Fc = [0.05; 0.05; 0.05];
F = B .* qd + Fc .* tanh(qd / 0.01);

% =========================
% DINÂMICA DIRETA
% qdd = inv(M)*(tau - C - G - F)
% =========================

qdd = M \ (tau(:) - C - G - F);

end

== matlab function sim_TCC_2024/Feedback Control with Iterative Learning Control MODEL B/PARCELA ILC PADRAO/ILC_COMUM1 ==
  data: Tspan input; Ts input; u output; error input; flag_Cycle output; t output; kp input; kd input; uf input; flag_HALF output
function [u, flag_Cycle, t,flag_HALF] = fcn(Tspan, Ts, error, kp, kd, uf)
persistent N samples_per_iter 
if isempty(N)
    N = round(Tspan/Ts); 
    samples_per_iter = N;
end

% -------------------------------------------------------------
% Memória persistente entre iterações
% -------------------------------------------------------------
persistent u_curr       % Comando de controle da iteração atual
persistent u_next       % Comando de controle da próxima iteração
persistent error_memory % Histórico de erros da iteração atual
persistent u_memory     % Histórico de torques da iteração atual
persistent k_iter       % Índice da iteração (ciclo)
persistent t_step       % Passo de tempo atual (1 até N)

if isempty(k_iter)
    k_iter = 1; 
    u_curr = zeros(1, N); 
    u_next = zeros(1, N);
    error_memory = zeros(1, N);
    u_memory = zeros(1, N);
    t_step = 1;
end

% -------------------------------------------------------------
% Lógica de Execução e Gravação (Sem saltar índices)
% -------------------------------------------------------------
% Aplica o torque calculado para o passo atual
u = u_curr(t_step);

% Grava perfeitamente os dados nas posições corretas (incluindo o passo 1)
error_memory(t_step) = error;
u_memory(t_step) = uf;

flag_Cycle = 0; % Por padrão, a flag de fim de ciclo é zero

if t_step <= samples_per_iter/2
    flag_HALF = 1;
else
    flag_HALF = 0;
end

% -------------------------------------------------------------
% Lógica de Aprendizagem (Executada exatamente no último ponto)
% -------------------------------------------------------------
if t_step == samples_per_iter
    
    e_k = error_memory;
    % Extrapolação suave: repete o último ponto em vez de colocar 0, evitando o degrau
    e_k1 = [error_memory(2:end), error_memory(end)];
    
    % Lei de atualização do ILC + PD Corrigida:
    % kp multiplica o erro atual (e_k). kd multiplica a derivada correta.
    u_next = u_memory + kp*e_k + kd*(e_k1 - e_k);
    % u_next = u_memory + kp/10*e_k;
    
    % Atualiza o perfil para o próximo ciclo
    u_curr = u_next; 
    k_iter = k_iter + 1; 
    
    t_step = 1; % Reseta o contador para começar o próximo ciclo no passo 1
    flag_Cycle = 1;   % Ativa a flag indicando fim de iteração
else
    t_step = t_step + 1; % Avança para o próximo passo de tempo
end

t = t_step;
end

== matlab function sim_TCC_2024/Feedback Control with Iterative Learning Control MODEL B/PARCELA ILC PADRAO/ILC_COMUM2 ==
  data: Tspan input; Ts input; u output; error input; flag output; t output; kp input; kd input; uf input
function [u, flag, t] = fcn(Tspan, Ts, error, kp, kd, uf)
persistent N samples_per_iter 
if isempty(N)
    N = round(Tspan/Ts); 
    samples_per_iter = N;
end

% -------------------------------------------------------------
% Memória persistente entre iterações
% -------------------------------------------------------------
persistent u_curr       % Comando de controle da iteração atual
persistent u_next       % Comando de controle da próxima iteração
persistent error_memory % Histórico de erros da iteração atual
persistent u_memory     % Histórico de torques da iteração atual
persistent k_iter       % Índice da iteração (ciclo)
persistent t_step       % Passo de tempo atual (1 até N)

if isempty(k_iter)
    k_iter = 1; 
    u_curr = zeros(1, N); 
    u_next = zeros(1, N);
    error_memory = zeros(1, N);
    u_memory = zeros(1, N);
    t_step = 1;
end

% -------------------------------------------------------------
% Lógica de Execução e Gravação (Sem saltar índices)
% -------------------------------------------------------------
% Aplica o torque calculado para o passo atual
u = u_curr(t_step);

% Grava perfeitamente os dados nas posições corretas (incluindo o passo 1)
error_memory(t_step) = error;
u_memory(t_step) = uf;

flag = 0; % Por padrão, a flag de fim de ciclo é zero

% -------------------------------------------------------------
% Lógica de Aprendizagem (Executada exatamente no último ponto)
% -------------------------------------------------------------
if t_step == samples_per_iter
    
    e_k = error_memory;
    % Extrapolação suave: repete o último ponto em vez de colocar 0, evitando o degrau
    e_k1 = [error_memory(2:end), error_memory(end)];
    
    % Lei de atualização do ILC + PD Corrigida:
    % kp multiplica o erro atual (e_k). kd multiplica a derivada correta.
    u_next = u_memory + kp*e_k + kd*(e_k1 - e_k);
    % u_next = u_memory + kp/10*e_k;
    
    % Atualiza o perfil para o próximo ciclo
    u_curr = u_next; 
    k_iter = k_iter + 1; 
    
    t_step = 1; % Reseta o contador para começar o próximo ciclo no passo 1
    flag = 1;   % Ativa a flag indicando fim de iteração
else
    t_step = t_step + 1; % Avança para o próximo passo de tempo
end

t = t_step;
end

== matlab function sim_TCC_2024/Equação de Corpo Rígido FeedForward3 ==
  data: q input; y output; qd input; qdd input
function y = CorpoRigido(q, qd, qdd)

% Parâmetros
l1 = 0.15;
l2 = 0.255;
l3 = 0.199;

m1 = 0.200;
m2 = 0.07576;
m3 = 0.07192;

g = 9.8;

theta2 = q(2);
theta3 = q(3);

v1 = qd(1);
v2 = qd(2);
v3 = qd(3);

% =========================
% MATRIZ DE INÉRCIA M(q)
% =========================

M11 = (1/2)*m1*l1^2 ...
    + (1/3)*m2*l2^2*cos(theta2)^2 ...
    + (1/3)*m3*l3^2*cos(theta2 + theta3)^2 ...
    + m3*l2^2*cos(theta2)^2 ...
    + m3*l2*l3*cos(theta2)*cos(theta2 + theta3);

M22 = (1/3)*m2*l2^2 ...
    + (1/3)*m3*l3^2 ...
    + m3*l2^2 ...
    + m3*l2*l3*cos(theta3);

M23 = (1/3)*m3*l3^2 ...
    + 0.5*m3*l2*l3*cos(theta3);

M33 = (1/3)*m3*l3^2;

M = [M11   0     0;
     0     M22   M23;
     0     M23   M33];

% =========================
% VETOR CORIOLIS/CENTRÍFUGO
% =========================

C1 = ( ...
    -(1/3)*m2*l2^2*sin(2*theta2) ...
    - m3*l2^2*sin(2*theta2) ...
    -(1/3)*m3*l3^2*sin(2*(theta2 + theta3)) ...
    - m3*l2*l3*sin(2*theta2 + theta3) ...
    )*v2*v1 ...
    + ( ...
    -(1/3)*m3*l3^2*sin(2*(theta2 + theta3)) ...
    - m3*l2*l3*cos(theta2)*sin(theta2 + theta3) ...
    )*v3*v1;

C2 = (-m3*l2*l3*sin(theta3))*v2*v3 ...
    + (-0.5*m3*l2*l3*sin(theta3))*v3^2 ...
    + ( ...
    (1/6)*m2*l2^2*sin(2*theta2) ...
    + (1/6)*m3*l3^2*sin(2*(theta2 + theta3)) ...
    + 0.5*m3*l2^2*sin(2*theta2) ...
    + 0.5*m3*l2*l3*sin(2*theta2 + theta3) ...
    )*v1^2;

C3 = (0.5*m3*l2*l3*sin(theta3))*v2^2 ...
    + ( ...
    (1/6)*m3*l3^2*sin(2*(theta2 + theta3)) ...
    + 0.5*m3*l2*l3*cos(theta2)*sin(theta2 + theta3) ...
    )*v1^2;

C = [C1; C2; C3];

% =========================
% VETOR GRAVITACIONAL G(q)
% =========================

G1 = 0;

G2 = 0.5*m2*g*l2*cos(theta2) ...
    + m3*g*l2*cos(theta2) ...
    + 0.5*m3*g*l3*cos(theta2 + theta3);

G3 = 0.5*m3*g*l3*cos(theta2 + theta3);

G = [G1; G2; G3];

% =========================
% TORQUE FINAL
% tau = M(q)qdd + C(q,qd) + G(q)
% =========================

tau = M*qdd(:) + C + G;

% Saída como vetor coluna
y = tau;

end

== matlab function sim_TCC_2024/Feedback Control with Iterative Learning Control MODEL B/MATLAB Function ==
  settings: sampleTime=0
  data: e0 output; q0 input; t0 output; Q0 input; qd0 input; QD0 input; q1 input; Q1 input; qd1 input; QD1 input; q2 input; Q2 input; qd2 input; QD2 input; t1 output; t2 output; Kp0 input; Kp1 input; Kp2 input; Kv0 input; Kv1 input; Kv2 input
function [e0,t0,t1,t2] = controle_IM(q0,Q0,qd0,QD0,q1,Q1,qd1,QD1,q2,Q2,qd2,QD2,Kp0,Kp1,Kp2,Kv0,Kv1,Kv2)


e0 = q0-Q0;
t0 = Kp0*(q0-Q0) + Kv0*(qd0-QD0);
t1 = Kp1*(q1-Q1) + Kv1*(qd1-QD1);
t2 = Kp2*(q2-Q2) + Kv2*(qd2-QD2);
end
